simulink model "simple_logic"  (R2020b)
settings: Solver=VariableStepAuto  StartTime=0.0  StopTime=10.0  RelTol=1e-3
values from neighbouring files (symbols this model uses):
  b = 0.1    [matlab.mat]
undefined symbols (not defined in the file or in its folder): a, c
libraries: simulink x3
settings Model: Creator=intel  LastModifiedBy=intel

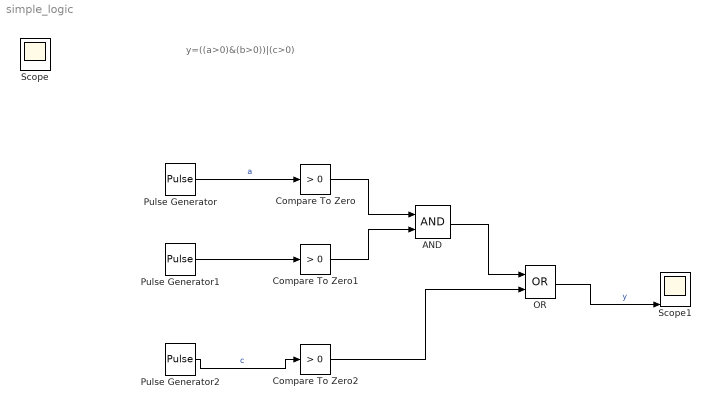
== system simple_logic ==
  note: y=((a>0)&(b>0))|(c>0)
  AND : Logic  AllPortsSameDT=off  OutDataTypeStr=boolean
  Compare To Zero : simulink/Logic and Bit Operations/Compare To Zero  relop=>  OutDataTypeStr=boolean
  Compare To Zero1 : simulink/Logic and Bit Operations/Compare To Zero  relop=>  OutDataTypeStr=boolean
  Compare To Zero2 : simulink/Logic and Bit Operations/Compare To Zero  relop=>  OutDataTypeStr=boolean
  OR : Logic  Operator=OR  AllPortsSameDT=off  OutDataTypeStr=boolean
  Pulse Generator : DiscretePulseGenerator  PulseType=Time based  Period=10  PulseWidth=20  PhaseDelay=a
  Pulse Generator1 : DiscretePulseGenerator  PulseType=Time based  Period=10  PulseWidth=20  PhaseDelay=b  VectorParams1D=off
  Pulse Generator2 : DiscretePulseGenerator  PulseType=Time based  Period=10  PulseWidth=20  PhaseDelay=c
  Scope1 : Scope  NumInputPorts=4
  Scope : Scope
  wires:
  Compare To Zero/1 -> AND/1
  Compare To Zero1/1 -> AND/2
  Compare To Zero2/1 -> OR/2
  AND/1 -> OR/1
  OR/1 -> Scope1/4  "y"
  Pulse Generator1/1 -> Compare To Zero1/1
  Pulse Generator2/1 -> Compare To Zero2/1  "c"
  Pulse Generator/1 -> Compare To Zero/1  "a"
